simulink model "SMC"  (R2023a)
settings: Solver=FixedStepAuto  StartTime=0.0  StopTime=200  RelTol=1e-3
settings Model: Creator=belov  LastModifiedBy=belov

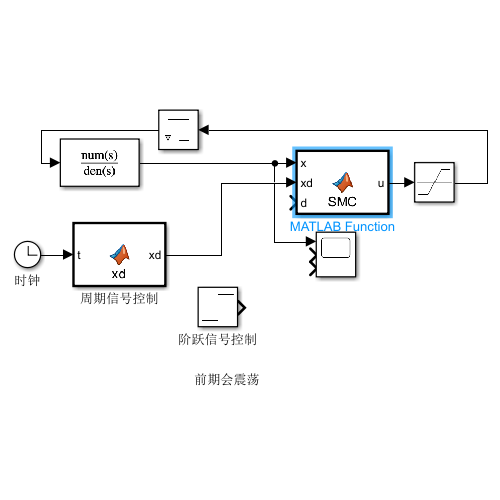
[thumbnail: Simulink's stored preview of the top-level diagram]
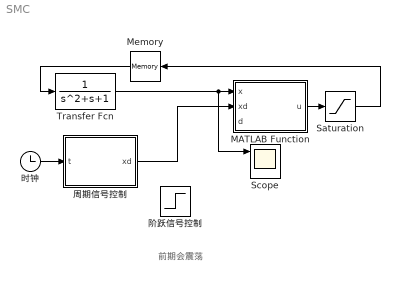
== system SMC ==
  note: 前期会震荡
  MATLAB Function : MATLAB Function  TreatAsAtomicUnit=on  SystemSampleTime=0.001
  Memory : Memory
  Saturation : Saturate  UpperLimit=5  LowerLimit=-5
  Scope : Scope  NumInputPorts=3
  Transfer Fcn : TransferFcn  Denominator=[1 1 1]
  周期信号控制 : MATLAB Function  TreatAsAtomicUnit=on  SystemSampleTime=0.001
  时钟 : Clock
  阶跃信号控制 : Step  SampleTime=0
  wires:
  时钟/1 -> 周期信号控制/1(t)
  Transfer Fcn/1 -> Scope/1, MATLAB Function/1(x)
  Memory/1 -> Transfer Fcn/1
  MATLAB Function/1(u) -> Saturation/1
  Saturation/1 -> Memory/1
  周期信号控制/1(xd) -> MATLAB Function/2(xd)

== matlab function SMC/MATLAB Function ==
  data: x input; u output; xd input; d input
function u = SMC(x, xd, d)
persistent acce xdlast elast;
tstep = 0.001;
b = 10;
k = 3;
c = 5;
D = 0.5;

if isempty(acce)
    acce = 0;
end
if isempty(elast)
    elast = 0;
end
if isempty(xdlast)
    xdlast = 0;
end

%%%% 一阶系统
% dxd = (xd - xdlast) / tstep;
% e = x - xd;
% acce = acce + (e + elast) * tstep / 2;
% s = e + c * acce;
% u = (dxd - c * e - k * s - D * sign(s)) / b;
% xdlast = xd;    
% elast = e;

%%%% 二阶系统
e = x - xd;
x2 = (e - elast) / tstep;
s = c * e + x2;
u = -k * sign(s) - c * x2 - k * s - d;
elast = e;

end

== matlab function SMC/周期信号控制 ==
  data: t input; xd output
function xd = xd(t)
xd = 4*cos(t / 10);
end
